simulink model "s3"  (Simulink 2.00)
settings: Solver=ode45  StartTime=0.0  StopTime=999999  MaxStep=10  RelTol=1e-3  AbsTol=1e-6
values from neighbouring files (symbols this model uses):
  Domega = 0    [M4.M]    (also in SET1.M; SET3A.M; SET3B.M; SET3C.M)
  H = 0.5*J_rotor*wbasem*wbasem/Sbase    [M1.M]    (also in M3.M; M4.M = 0.3; SET1.M = 3.77; SET3A.M = 3)
  Psido = xls*(-Ido) + Psiado    [M1.M]    (also in M3.M; M4.M = Psiado; M5.M)
  Psifo = xplf*Ifo + Psiado    [M1.M]    (also in M3.M; M5.M = (xpr2c+xpr1c+xp1c)*Ifo + Psiado)
  Psikdo = Psiado    [M1.M]    (also in M3.M; M4.M)
  Psikqo = Psiaqo    [M1.M]    (also in M3.M; M4.M = 0)
  Psiqo = xls*(-Iqo) + Psiaqo    [M1.M]    (also in M3.M; M4.M = 0; M5.M)
  rpf = rpf/Zbase    [M1.M]    (also in M3.M; SET3A.M = 0.00112; SET3B.M = 0.00109)
  rpkd = rpkd/Zbase    [M1.M]    (also in M3.M; M4.M = 0.054)
  rpkq = rpkq/Zbase    [M1.M]    (also in M3.M; M4.M = 0.108)
  rs = rs/Zbase    [M1.M]    (also in M3.M; M4.M = 0.017; SET1.M = 0.0048; SET3A.M = 0.004)
  wb = wbase    [M1.M]    (also in M3.M; M4.M = 376.991118431; M5.M)
  xls = xls/Zbase    [M1.M]    (also in M3.M; M4.M = 0.065; SET1.M = 0.215; SET3A.M = 0.19)
  xmd = xmd/Zbase    [M1.M]    (also in M3.M; M4.M = 0.478; SET3A.M = 1.7; SET3B.M = 1.7)
  xMD = (1/xls + 1/xmd + 1/xplf + 1/xplkd)^(-1)    [M1.M]    (also in M3.M; M4.M = 0.0399162984447; M5.M = (1/xls + 1/xmd + bsum)^(-1))
  xMQ = (1/xls + 1/xmq + 1/xplkq)^(-1)    [M1.M]    (also in M3.M; M4.M = 0.0417714348384; M5.M = (1/xls + 1/xmq + 1/xplkq3 + 1/xplkq2 + 1/xplkq1)^(-1))
  xplf = xplf/Zbase    [M1.M]    (also in M3.M)
  xplkd = xplkd/Zbase    [M1.M]    (also in M3.M; M4.M = 0.132)
  xplkq = xplkq/Zbase    [M1.M]    (also in M3.M; M4.M = 0.132)
settings Model: SaveTime=off  SaveOutput=off  ConsistencyChecking=off

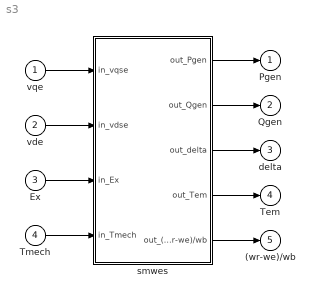
== system s3 ==
  vqe : Inport  Port=1  PortWidth=-1  SampleTime=-1
  vde : Inport  Port=2  PortWidth=-1  SampleTime=-1
  Ex : Inport  Port=3  PortWidth=-1  SampleTime=-1
  Tmech : Inport  Port=4  PortWidth=-1  SampleTime=-1
  smwes : Subsystem
  Pgen : Outport  Port=1  InitialOutput=0
  Qgen : Outport  Port=2  InitialOutput=0
  delta : Outport  Port=3  InitialOutput=0
  Tem : Outport  Port=4  InitialOutput=0
  (wr-we)/wb : Outport  Port=5  InitialOutput=0
  wires:
  Tmech/1 -> smwes/4(in_Tmech)
  smwes/1(out_Pgen) -> Pgen/1
  smwes/2(out_Qgen) -> Qgen/1
  smwes/3(out_delta) -> delta/1
  Ex/1 -> smwes/3(in_Ex)
  vqe/1 -> smwes/1(in_vqse)
  vde/1 -> smwes/2(in_vdse)
  smwes/4(out_Tem) -> Tem/1
  smwes/5(out_(wr-we)/wb) -> (wr-we)/wb/1

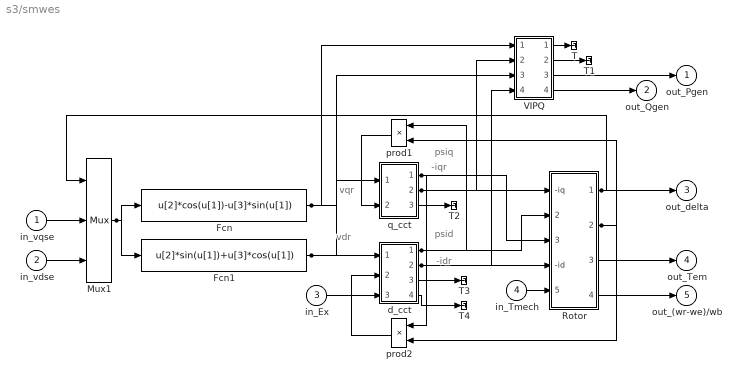
== system s3/smwes ==
  note: vdr
  note: vqr
  note: -iqr
  note: psid
  note: psiq
  note: -idr
  in_vqse : Inport  Port=1  PortWidth=-1  SampleTime=-1
  in_vdse : Inport  Port=2  PortWidth=-1  SampleTime=-1
  in_Ex : Inport  Port=3  PortWidth=-1  SampleTime=-1
  in_Tmech : Inport  Port=4  PortWidth=-1  SampleTime=-1
  Fcn : Fcn  Expr=u[2]*cos(u[1])-u[3]*sin(u[1])
  Fcn1 : Fcn  Expr=u[2]*sin(u[1])+u[3]*cos(u[1])
  Mux1 : Mux  Inputs=3
  Rotor : Subsystem
  T{,1..4} (5 alike) : Terminator
  VIPQ : Subsystem
  d_cct : Subsystem
  prod1 : Product  Orientation=left  Inputs=2
  prod2 : Product  Orientation=left  Inputs=2
  q_cct : Subsystem
  out_Pgen : Outport  Port=1  InitialOutput=0
  out_Qgen : Outport  Port=2  InitialOutput=0
  out_delta : Outport  Port=3  InitialOutput=0
  out_Tem : Outport  Port=4  InitialOutput=0
  out_(wr-we)/wb : Outport  Port=5  InitialOutput=0
  wires:
  Rotor/2("wr/wb ") -> prod1/2, prod2/2
  q_cct/1(Out_psiq) -> prod2/1, Rotor/3(psiq)
  d_cct/1(Out_psid) -> prod1/1, Rotor/2("psid ")
  prod2/1 -> d_cct/2(In_wrpsiq)
  Rotor/3(Tem) -> out_Tem/1
  in_Ex/1 -> d_cct/3(In_Ef)
  Rotor/4((wr-we)/wb) -> out_(wr-we)/wb/1
  in_Tmech/1 -> Rotor/5(Tmech)
  in_vqse/1 -> Mux1/2
  in_vdse/1 -> Mux1/3
  Rotor/1(delta) -> out_delta/1, Mux1/1
  Mux1/1 -> Fcn/1, Fcn1/1
  q_cct/2(Out_-iq) -> Rotor/1(-iq), VIPQ/2(-iqr)
  d_cct/2(Out_-id) -> Rotor/4(-id), VIPQ/4(-idr)
  Fcn/1 -> q_cct/1(In_vqr), VIPQ/1(vqr)
  Fcn1/1 -> d_cct/1(In_vdr), VIPQ/3(vdr)
  VIPQ/3(Pgen) -> out_Pgen/1
  VIPQ/4(Qgen) -> out_Qgen/1
  prod1/1 -> q_cct/2(In_wrpsid)
  VIPQ/1(Out_|Vt|) -> T/1
  q_cct/3(Out_psimq) -> T2/1
  d_cct/3(Out_psimd) -> T3/1
  d_cct/4(Out_ipf) -> T4/1
  VIPQ/2(Out_|It|) -> T1/1

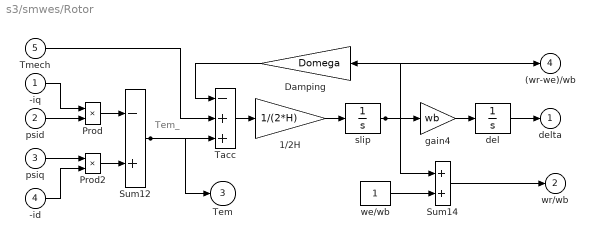
== system s3/smwes/Rotor ==
  note: Tem_
  -iq : Inport  Port=1  PortWidth=-1  SampleTime=-1
  "psid " : Inport  Port=2  PortWidth=-1  SampleTime=-1
  psiq : Inport  Port=3  PortWidth=-1  SampleTime=-1
  -id : Inport  Port=4  PortWidth=-1  SampleTime=-1
  Tmech : Inport  Port=5  PortWidth=-1  SampleTime=-1
  1/2H : Gain  Gain=1/(2*H)
  Damping : Gain  Orientation=left  Gain=Domega
  Prod : Product  Inputs=2
  Prod2 : Product  Inputs=2
  Sum12 : Sum  Inputs=-+
  Sum14 : Sum  Inputs=++
  Tacc : Sum  Inputs=-++
  del : Integrator  ExternalReset=none  InitialConditionSource=internal  InitialCondition=0  LimitOutput=off  UpperSaturationLimit=inf  LowerSaturationLimit=-inf  ShowSaturationPort=off  ShowStatePort=off  AbsoluteTolerance=auto
  gain4 : Gain  Gain=wb
  slip : Integrator  ExternalReset=none  InitialConditionSource=internal  InitialCondition=0  LimitOutput=off  UpperSaturationLimit=inf  LowerSaturationLimit=-inf  ShowSaturationPort=off  ShowStatePort=off  AbsoluteTolerance=auto
  we/wb : Constant  Value=1
  delta : Outport  Port=1  InitialOutput=0
  "wr/wb " : Outport  Port=2  InitialOutput=0
  Tem : Outport  Port=3  InitialOutput=0
  (wr-we)/wb : Outport  Port=4  InitialOutput=0
  wires:
  Damping/1 -> Tacc/1
  gain4/1 -> del/1
  Prod2/1 -> Sum12/2
  1/2H/1 -> slip/1
  we/wb/1 -> Sum14/2
  Tacc/1 -> 1/2H/1
  Prod/1 -> Sum12/1
  -iq/1 -> Prod/1
  "psid "/1 -> Prod/2
  psiq/1 -> Prod2/1
  -id/1 -> Prod2/2
  Sum14/1 -> "wr/wb "/1
  Sum12/1 -> Tacc/3, Tem/1
  slip/1 -> gain4/1, Sum14/1, Damping/1, (wr-we)/wb/1
  Tmech/1 -> Tacc/2
  del/1 -> delta/1

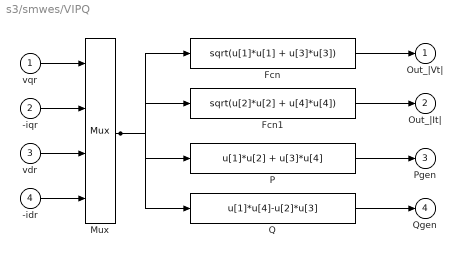
== system s3/smwes/VIPQ ==
  vqr : Inport  Port=1  PortWidth=-1  SampleTime=-1
  -iqr : Inport  Port=2  PortWidth=-1  SampleTime=-1
  vdr : Inport  Port=3  PortWidth=-1  SampleTime=-1
  -idr : Inport  Port=4  PortWidth=-1  SampleTime=-1
  Fcn : Fcn  Expr=sqrt(u[1]*u[1] + u[3]*u[3])
  Fcn1 : Fcn  Expr=sqrt(u[2]*u[2] + u[4]*u[4])
  Mux : Mux  Inputs=4
  P : Fcn  Expr=u[1]*u[2] + u[3]*u[4]
  Q : Fcn  Expr=u[1]*u[4]-u[2]*u[3]
  Out_|Vt| : Outport  Port=1  InitialOutput=0
  Out_|It| : Outport  Port=2  InitialOutput=0
  Pgen : Outport  Port=3  InitialOutput=0
  Qgen : Outport  Port=4  InitialOutput=0
  wires:
  vqr/1 -> Mux/1
  -iqr/1 -> Mux/2
  vdr/1 -> Mux/3
  -idr/1 -> Mux/4
  P/1 -> Pgen/1
  Q/1 -> Qgen/1
  Mux/1 -> P/1, Q/1, Fcn/1, Fcn1/1
  Fcn1/1 -> Out_|It|/1
  Fcn/1 -> Out_|Vt|/1

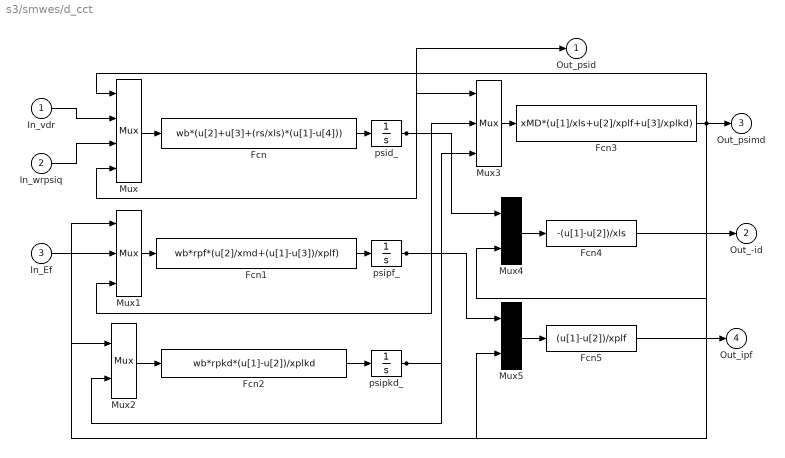
== system s3/smwes/d_cct ==
  In_vdr : Inport  Port=1  PortWidth=-1  SampleTime=-1
  In_wrpsiq : Inport  Port=2  PortWidth=-1  SampleTime=-1
  In_Ef : Inport  Port=3  PortWidth=-1  SampleTime=-1
  Fcn : Fcn  Expr=wb*(u[2]+u[3]+(rs/xls)*(u[1]-u[4]))
  Fcn1 : Fcn  Expr=wb*rpf*(u[2]/xmd+(u[1]-u[3])/xplf)
  Fcn2 : Fcn  Expr=wb*rpkd*(u[1]-u[2])/xplkd
  Fcn3 : Fcn  Expr=xMD*(u[1]/xls+u[2]/xplf+u[3]/xplkd)
  Fcn4 : Fcn  Expr=-(u[1]-u[2])/xls
  Fcn5 : Fcn  Expr=(u[1]-u[2])/xplf
  Mux : Mux  Inputs=4
  Mux1 : Mux  Inputs=3
  Mux2 : Mux  Inputs=2
  Mux3 : Mux  Inputs=3
  Mux4 : Mux  Inputs=2
  Mux5 : Mux  Inputs=2
  psid_ : Integrator  ExternalReset=none  InitialConditionSource=internal  InitialCondition=Psido  LimitOutput=off  UpperSaturationLimit=inf  LowerSaturationLimit=-inf  ShowSaturationPort=off  ShowStatePort=off  AbsoluteTolerance=auto
  psipf_ : Integrator  ExternalReset=none  InitialConditionSource=internal  InitialCondition=Psifo  LimitOutput=off  UpperSaturationLimit=inf  LowerSaturationLimit=-inf  ShowSaturationPort=off  ShowStatePort=off  AbsoluteTolerance=auto
  psipkd_ : Integrator  ExternalReset=none  InitialConditionSource=internal  InitialCondition=Psikdo  LimitOutput=off  UpperSaturationLimit=inf  LowerSaturationLimit=-inf  ShowSaturationPort=off  ShowStatePort=off  AbsoluteTolerance=auto
  Out_psid : Outport  Port=1  InitialOutput=0
  Out_-id : Outport  Port=2  InitialOutput=0
  Out_psimd : Outport  Port=3  InitialOutput=0
  Out_ipf : Outport  Port=4  InitialOutput=0
  wires:
  In_wrpsiq/1 -> Mux/3
  In_vdr/1 -> Mux/2
  Mux/1 -> Fcn/1
  Fcn/1 -> psid_/1
  Mux1/1 -> Fcn1/1
  Fcn1/1 -> psipf_/1
  In_Ef/1 -> Mux1/2
  Mux2/1 -> Fcn2/1
  Fcn2/1 -> psipkd_/1
  psid_/1 -> Mux/4, Mux3/1, Mux4/1, Out_psid/1
  psipf_/1 -> Mux1/3, Mux3/2, Mux5/1
  psipkd_/1 -> Mux2/2, Mux3/3
  Mux3/1 -> Fcn3/1
  Mux4/1 -> Fcn4/1
  Mux5/1 -> Fcn5/1
  Fcn3/1 -> Mux5/2, Mux4/2, Mux2/1, Mux1/1, Mux/1, Out_psimd/1
  Fcn4/1 -> Out_-id/1
  Fcn5/1 -> Out_ipf/1

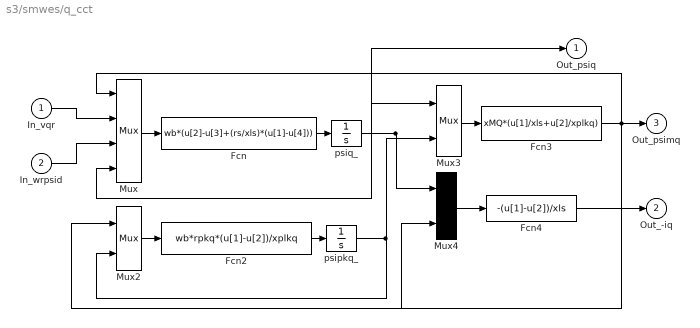
== system s3/smwes/q_cct ==
  In_vqr : Inport  Port=1  PortWidth=-1  SampleTime=-1
  In_wrpsid : Inport  Port=2  PortWidth=-1  SampleTime=-1
  Fcn : Fcn  Expr=wb*(u[2]-u[3]+(rs/xls)*(u[1]-u[4]))
  Fcn2 : Fcn  Expr=wb*rpkq*(u[1]-u[2])/xplkq
  Fcn3 : Fcn  Expr=xMQ*(u[1]/xls+u[2]/xplkq)
  Fcn4 : Fcn  Expr=-(u[1]-u[2])/xls
  Mux : Mux  Inputs=4
  Mux2 : Mux  Inputs=2
  Mux3 : Mux  Inputs=2
  Mux4 : Mux  Inputs=2
  psipkq_ : Integrator  ExternalReset=none  InitialConditionSource=internal  InitialCondition=Psikqo  LimitOutput=off  UpperSaturationLimit=inf  LowerSaturationLimit=-inf  ShowSaturationPort=off  ShowStatePort=off  AbsoluteTolerance=auto
  psiq_ : Integrator  ExternalReset=none  InitialConditionSource=internal  InitialCondition=Psiqo  LimitOutput=off  UpperSaturationLimit=inf  LowerSaturationLimit=-inf  ShowSaturationPort=off  ShowStatePort=off  AbsoluteTolerance=auto
  Out_psiq : Outport  Port=1  InitialOutput=0
  Out_-iq : Outport  Port=2  InitialOutput=0
  Out_psimq : Outport  Port=3  InitialOutput=0
  wires:
  In_wrpsid/1 -> Mux/3
  In_vqr/1 -> Mux/2
  Mux/1 -> Fcn/1
  Fcn/1 -> psiq_/1
  Mux2/1 -> Fcn2/1
  Fcn2/1 -> psipkq_/1
  psiq_/1 -> Mux/4, Mux3/1, Mux4/1, Out_psiq/1
  psipkq_/1 -> Mux2/2, Mux3/2
  Mux3/1 -> Fcn3/1
  Mux4/1 -> Fcn4/1
  Fcn3/1 -> Mux4/2, Mux2/1, Mux/1, Out_psimq/1
  Fcn4/1 -> Out_-iq/1
